simulink model "Water_Treatment_Plant"  (R2024b)
settings: Solver=VariableStepAuto  StartTime=0.0  StopTime=10.0  RelTol=1e-3
settings Model: Creator=jakeo  LastModifiedBy=jakeo

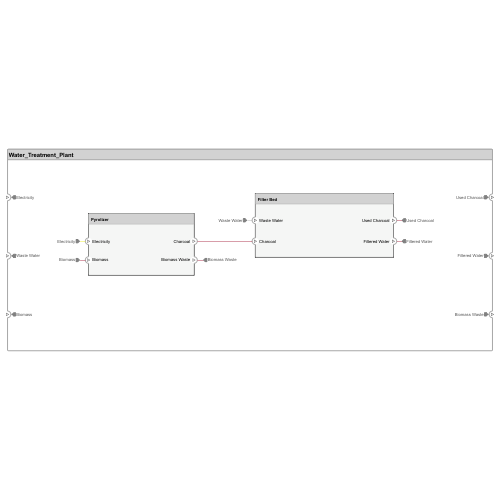
[thumbnail: Simulink's stored preview of the top-level diagram]
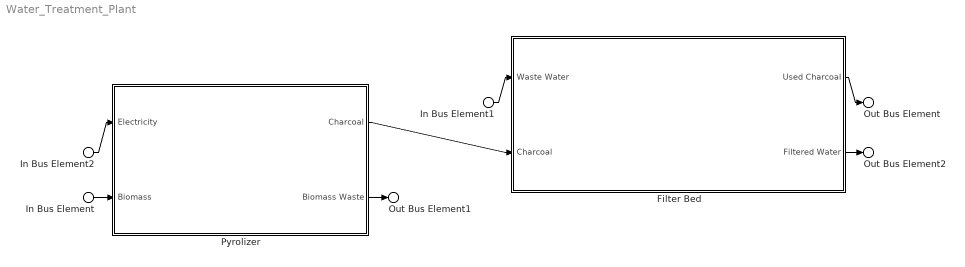
== system Water_Treatment_Plant ==
  In Bus Element2 : Inport  PortName=Electricity
  In Bus Element1 : Inport  Port=2  PortName=Waste Water
  In Bus Element : Inport  Port=3  PortName=Biomass
  Filter Bed : Subsystem
      settings: PortSchema="{\"entries\":[{\"content\":{\"headerSize\":26,\"margin\":15,\"minimumSpacing\":25,\"sides\":[{\"content\":{\"connectorIds\":[\"In1\",\"In2\"]},\"type\":\"ConnectorPlacement.EquallySpacedRectSide\",\"uuid\":\"3794ce98-e5af-4a84-b3ea-0b1fb9c3c967\"},{\"content\":{\"connectorIds\":[\"Out1\",\"Out2\"],\"side\":\"RIGHT\"},\"type\":\"ConnectorPlacement.EquallySpacedRectSide\",\"uuid\":\"33785edc-c7e9-47e5-a30e-8a8341eb0e2e\"},{\"content\":{\"side\":\"TOP\"},\"type\":\"ConnectorPlacement.EquallySpacedRectSide\",\"uuid\":\"d59b4e74-597d-4de8-8eb7-892a86f0c4f5\"}]},\"type\":\"ConnectorPlacement.EquallySpacedConnector\",\"uuid\":\"b145d864-7188-4e8b-81d2-38fb7cb7b9ed\"}],\"packageUris\":[\"http://schema.mathworks.com/mf0/Connector/R2020b\"],\"version\":\"1.0\"}"
  Pyrolizer : Subsystem
      settings: PortSchema="{\"entries\":[{\"content\":{\"headerSize\":26,\"margin\":15,\"minimumSpacing\":25,\"sides\":[{\"content\":{\"connectorIds\":[\"In1\",\"In2\"]},\"type\":\"ConnectorPlacement.EquallySpacedRectSide\",\"uuid\":\"3794ce98-e5af-4a84-b3ea-0b1fb9c3c967\"},{\"content\":{\"connectorIds\":[\"Out2\",\"Out1\"],\"side\":\"RIGHT\"},\"type\":\"ConnectorPlacement.EquallySpacedRectSide\",\"uuid\":\"33785edc-c7e9-47e5-a30e-8a8341eb0e2e\"},{\"content\":{\"side\":\"TOP\"},\"type\":\"ConnectorPlacement.EquallySpacedRectSide\",\"uuid\":\"d59b4e74-597d-4de8-8eb7-892a86f0c4f5\"},{\"content\":{\"side\":\"BOTTOM\"},\"type\":\"ConnectorPlacement.EquallySpacedRectSide\",\"uuid\":\"32d95b18-0871-4c3f-842c-e1f6da212166\"}]},\"type\":\"ConnectorPlacement.EquallySpacedConnector\",\"uuid\":\"b145d864-7188-4e8b-81d2-38fb7cb7b9ed\"}],\"packageUris\":[\"http://schema.mathworks.com/mf0/Connector/R2020b\"],\"version\":\"1.0\"}"
  Out Bus Element : Outport  PortName=Used Charcoal
  Out Bus Element2 : Outport  Port=2  PortName=Filtered Water
  Out Bus Element1 : Outport  Port=3  PortName=Biomass Waste
  wires:
  In Bus Element/1 -> Pyrolizer/2(Biomass)
  Pyrolizer/2(Charcoal) -> Filter Bed/2(Charcoal)
  Filter Bed/1(Used Charcoal) -> Out Bus Element/1
  Pyrolizer/1(Biomass Waste) -> Out Bus Element1/1
  In Bus Element1/1 -> Filter Bed/1(Waste Water)
  Filter Bed/2(Filtered Water) -> Out Bus Element2/1
  In Bus Element2/1 -> Pyrolizer/1(Electricity)

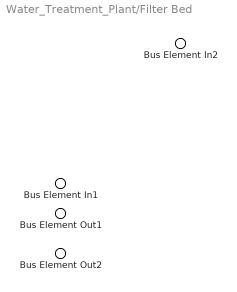
== system Water_Treatment_Plant/Filter Bed ==
  Bus Element In2 : Inport  PortName=Waste Water
  Bus Element In1 : Inport  Port=2  PortName=Charcoal
  Bus Element Out1 : Outport  PortName=Used Charcoal
  Bus Element Out2 : Outport  Port=2  PortName=Filtered Water

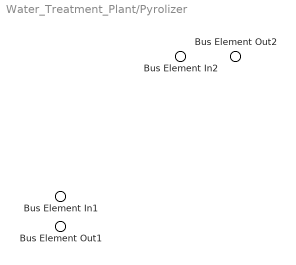
== system Water_Treatment_Plant/Pyrolizer ==
  Bus Element In2 : Inport  PortName=Electricity
  Bus Element In1 : Inport  Port=2  PortName=Biomass
  Bus Element Out2 : Outport  PortName=Biomass Waste
  Bus Element Out1 : Outport  Port=2  PortName=Charcoal
